simulink library "csc_wpc_watchpoint_collection_lib"  (R2015b)
settings: Solver=VariableStepAuto  StartTime=0.0  StopTime=10.0  RelTol=1e-3
undefined symbols (not defined in the file or in its folder): enum_mode, enum_submode
libraries: csu_ewp_evaluate_wp_lib x14, util_info_lib x1
settings Model: Creator=Mark Agbayani  LastModifiedBy=jimkaidy

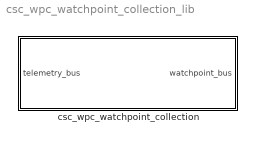
== system csc_wpc_watchpoint_collection_lib ==
  csc_wpc_watchpoint_collection : Subsystem
      mask Display: color('blue');text(0.05, 0.02, 'MoonEx', 'HorizontalAlignment', 'Left', 'VerticalAlignment', 'Bottom');color('red');text(0.95, 0.02, 'Autogenerated', 'HorizontalAlignment', 'Right', 'VerticalAlignment', 'Bottom');

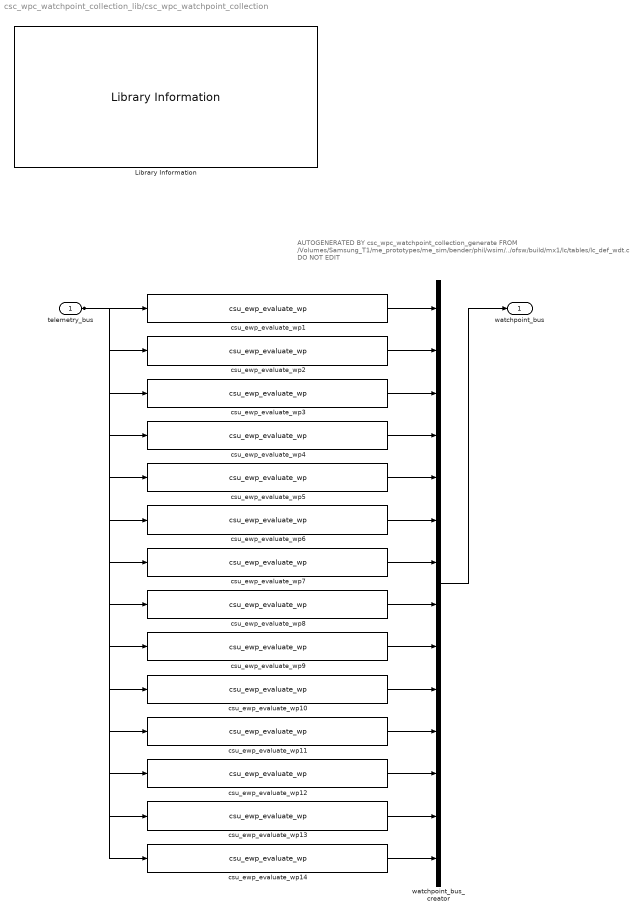
== system csc_wpc_watchpoint_collection_lib/csc_wpc_watchpoint_collection ==
  note: AUTOGENERATED BY csc_wpc_watchpoint_collection_generate FROM
      | /Volumes/Samsung_T1/me_prototypes/me_sim/bender/phil/wsim/../ofsw/build/mx1/lc/tables/lc_def_wdt.c
      | DO NOT EDIT
  telemetry_bus : Inport
  Library Information : util_info_lib/Library Information  owner='escrane'
  csu_ewp_evaluate_wp1 : csu_ewp_evaluate_wp_lib/csu_ewp_evaluate_wp  wp_id=1  signal_name=cmp_bus_msg.mode  signal_index=1  comparison_value=uint8(enum_mode.startup)  comparison_type===  bitmask_value=0
  csu_ewp_evaluate_wp10 : csu_ewp_evaluate_wp_lib/csu_ewp_evaluate_wp  wp_id=10  signal_name=cnt_bus_msg.main_thruster_cmd  signal_index=1  comparison_value=0  comparison_type===  bitmask_value=0
  csu_ewp_evaluate_wp11 : csu_ewp_evaluate_wp_lib/csu_ewp_evaluate_wp  wp_id=11  signal_name=cmp_bus_msg.submode  signal_index=1  comparison_value=uint8(enum_submode.landing_targeting)  comparison_type===  bitmask_value=0
  csu_ewp_evaluate_wp12 : csu_ewp_evaluate_wp_lib/csu_ewp_evaluate_wp  wp_id=12  signal_name=cmp_bus_msg.mode  signal_index=1  comparison_value=uint8(enum_mode.braking)  comparison_type===  bitmask_value=0
  csu_ewp_evaluate_wp13 : csu_ewp_evaluate_wp_lib/csu_ewp_evaluate_wp  wp_id=13  signal_name=cmp_bus_msg.submode  signal_index=1  comparison_value=uint8(enum_submode.landing_hold)  comparison_type===  bitmask_value=0
  csu_ewp_evaluate_wp14 : csu_ewp_evaluate_wp_lib/csu_ewp_evaluate_wp  wp_id=14  signal_name=gdn_bus_msg.burn_complete  signal_index=1  comparison_value=1  comparison_type===  bitmask_value=0
  csu_ewp_evaluate_wp2 : csu_ewp_evaluate_wp_lib/csu_ewp_evaluate_wp  wp_id=2  signal_name=cmp_bus_msg.mode  signal_index=1  comparison_value=uint8(enum_mode.landing)  comparison_type===  bitmask_value=0
  csu_ewp_evaluate_wp3 : csu_ewp_evaluate_wp_lib/csu_ewp_evaluate_wp  wp_id=3  signal_name=cmp_bus_msg.submode  signal_index=1  comparison_value=uint8(enum_submode.landing_terminal)  comparison_type===  bitmask_value=0
  csu_ewp_evaluate_wp4 : csu_ewp_evaluate_wp_lib/csu_ewp_evaluate_wp  wp_id=4  signal_name=gdn_bus_msg.hold_complete  signal_index=1  comparison_value=1  comparison_type===  bitmask_value=0
  csu_ewp_evaluate_wp5 : csu_ewp_evaluate_wp_lib/csu_ewp_evaluate_wp  wp_id=5  signal_name=gdn_bus_msg.targeting_complete  signal_index=1  comparison_value=0  comparison_type=~=  bitmask_value=0
  csu_ewp_evaluate_wp6 : csu_ewp_evaluate_wp_lib/csu_ewp_evaluate_wp  wp_id=6  signal_name=cmp_bus_msg.mode  signal_index=1  comparison_value=uint8(enum_mode.surface)  comparison_type===  bitmask_value=0
  csu_ewp_evaluate_wp7 : csu_ewp_evaluate_wp_lib/csu_ewp_evaluate_wp  wp_id=7  signal_name=est_bus_msg.landed  signal_index=1  comparison_value=0  comparison_type=~=  bitmask_value=0
  csu_ewp_evaluate_wp8 : csu_ewp_evaluate_wp_lib/csu_ewp_evaluate_wp  wp_id=8  signal_name=cmp_bus_msg.takeoff_enable  signal_index=1  comparison_value=1  comparison_type===  bitmask_value=0
  csu_ewp_evaluate_wp9 : csu_ewp_evaluate_wp_lib/csu_ewp_evaluate_wp  wp_id=9  signal_name=cnt_bus_msg.main_thruster_cmd  signal_index=1  comparison_value=0  comparison_type=~=  bitmask_value=0
  watchpoint_bus_creator : BusCreator  Inputs=14
  watchpoint_bus : Outport
  wires:
  watchpoint_bus_creator/1 -> watchpoint_bus/1
  telemetry_bus/1 -> csu_ewp_evaluate_wp1/1, csu_ewp_evaluate_wp2/1, csu_ewp_evaluate_wp3/1, csu_ewp_evaluate_wp4/1, csu_ewp_evaluate_wp5/1, csu_ewp_evaluate_wp6/1, csu_ewp_evaluate_wp7/1, csu_ewp_evaluate_wp8/1, csu_ewp_evaluate_wp9/1, csu_ewp_evaluate_wp10/1, csu_ewp_evaluate_wp11/1, csu_ewp_evaluate_wp12/1, csu_ewp_evaluate_wp13/1, csu_ewp_evaluate_wp14/1
  csu_ewp_evaluate_wp1/1 -> watchpoint_bus_creator/1
  csu_ewp_evaluate_wp2/1 -> watchpoint_bus_creator/2
  csu_ewp_evaluate_wp3/1 -> watchpoint_bus_creator/3
  csu_ewp_evaluate_wp4/1 -> watchpoint_bus_creator/4
  csu_ewp_evaluate_wp5/1 -> watchpoint_bus_creator/5
  csu_ewp_evaluate_wp6/1 -> watchpoint_bus_creator/6
  csu_ewp_evaluate_wp7/1 -> watchpoint_bus_creator/7
  csu_ewp_evaluate_wp8/1 -> watchpoint_bus_creator/8
  csu_ewp_evaluate_wp9/1 -> watchpoint_bus_creator/9
  csu_ewp_evaluate_wp10/1 -> watchpoint_bus_creator/10
  csu_ewp_evaluate_wp11/1 -> watchpoint_bus_creator/11
  csu_ewp_evaluate_wp12/1 -> watchpoint_bus_creator/12
  csu_ewp_evaluate_wp13/1 -> watchpoint_bus_creator/13
  csu_ewp_evaluate_wp14/1 -> watchpoint_bus_creator/14
